simulink model "c09f12_01_avn"  (R2012b)
settings: Solver=ode45  StartTime=0.0  StopTime="(2^(7+2))  * (2^8)"  RelTol=1e-3
undefined symbols (not defined in the file): Down, pfb_coeff_gen_calc, Up, xlipgetpartsetting
libraries: xbsIndex_r4 x7041, casper_library_misc x193, xps_library x58, casper_library_delays x50, simulink x16, dspsigops x12, casper_library_flow_control x5, xbsReplacements_r4 x4, casper_library_ffts_twiddle x2, casper_library_multipliers x2, casper_library_reorder x1
(part 4 of 77)

== system c09f12_01_avn/decat0 ==
  In1 : Inport
  Reinterpret{1..4} (4 alike) : xbsIndex_r4/Reinterpret  force_arith_type=on  arith_type="Signed  (2's comp)"  force_bin_pt=on  bin_pt=0  block_type=reinterpret
      settings: infoedit="Changes signal type without altering the binary representation.   You can changed the signal between signed and unsigned, and relocate the binary point.<br><br>Hardware notes: In hardware this block costs nothing.<br><br>Example:  Suppose the input is 6 bits wide, signed, with 2 fractional bits, and the output is forced to unsigned with 0 fractional bits.  Then an input of -2.0 (1110.00 in binary 2's complement) becomes an output of 56 (111000 in binary)."  block_version=10.1.3
  Slice15 : xbsIndex_r4/Slice  nbits=8  boolean_output=off  mode=Lower Bit Location + Width  bit1=0  base1=MSB of Input  bit0=8  base0=LSB of Input  dbl_ovrd=off  block_type=slice
      settings: infoedit="Extracts a given range of bits from each input sample and presents it at the output.  The output type is ordinarily unsigned with binary point at zero, but can be Boolean when the slice is one bit wide.<P><P>Hardware notes: In hardware this block costs nothing."  block_version=10.1.3
  Slice16 : xbsIndex_r4/Slice  nbits=8  boolean_output=off  mode=Lower Bit Location + Width  bit1=0  base1=MSB of Input  bit0=16  base0=LSB of Input  dbl_ovrd=off  block_type=slice
      settings: infoedit="Extracts a given range of bits from each input sample and presents it at the output.  The output type is ordinarily unsigned with binary point at zero, but can be Boolean when the slice is one bit wide.<P><P>Hardware notes: In hardware this block costs nothing."  block_version=10.1.3
  Slice17 : xbsIndex_r4/Slice  nbits=8  boolean_output=off  mode=Lower Bit Location + Width  bit1=0  base1=MSB of Input  bit0=24  base0=LSB of Input  dbl_ovrd=off  block_type=slice
      settings: infoedit="Extracts a given range of bits from each input sample and presents it at the output.  The output type is ordinarily unsigned with binary point at zero, but can be Boolean when the slice is one bit wide.<P><P>Hardware notes: In hardware this block costs nothing."  block_version=10.1.3
  Slice9 : xbsIndex_r4/Slice  nbits=8  boolean_output=off  mode=Lower Bit Location + Width  bit1=0  base1=MSB of Input  bit0=0  base0=LSB of Input  dbl_ovrd=off  block_type=slice
      settings: infoedit="Extracts a given range of bits from each input sample and presents it at the output.  The output type is ordinarily unsigned with binary point at zero, but can be Boolean when the slice is one bit wide.<P><P>Hardware notes: In hardware this block costs nothing."  block_version=10.1.3
  Out1 : Outport
  Out2 : Outport  Port=2
  Out3 : Outport  Port=3
  Out4 : Outport  Port=4
  wires:
  Reinterpret4/1 -> Out4/1
  Reinterpret3/1 -> Out3/1
  Reinterpret1/1 -> Out2/1
  Reinterpret2/1 -> Out1/1
  Slice9/1 -> Reinterpret4/1
  Slice15/1 -> Reinterpret3/1
  Slice16/1 -> Reinterpret1/1
  Slice17/1 -> Reinterpret2/1
  In1/1 -> Slice15/1, Slice9/1, Slice16/1, Slice17/1

== system c09f12_01_avn/decat1 ==
  In1 : Inport
  Reinterpret{1..4} (4 alike) : xbsIndex_r4/Reinterpret  force_arith_type=on  arith_type="Signed  (2's comp)"  force_bin_pt=on  bin_pt=0  block_type=reinterpret
      settings: infoedit="Changes signal type without altering the binary representation.   You can changed the signal between signed and unsigned, and relocate the binary point.<br><br>Hardware notes: In hardware this block costs nothing.<br><br>Example:  Suppose the input is 6 bits wide, signed, with 2 fractional bits, and the output is forced to unsigned with 0 fractional bits.  Then an input of -2.0 (1110.00 in binary 2's complement) becomes an output of 56 (111000 in binary)."  block_version=10.1.3
  Slice15 : xbsIndex_r4/Slice  nbits=8  boolean_output=off  mode=Lower Bit Location + Width  bit1=0  base1=MSB of Input  bit0=8  base0=LSB of Input  dbl_ovrd=off  block_type=slice
      settings: infoedit="Extracts a given range of bits from each input sample and presents it at the output.  The output type is ordinarily unsigned with binary point at zero, but can be Boolean when the slice is one bit wide.<P><P>Hardware notes: In hardware this block costs nothing."  block_version=10.1.3
  Slice16 : xbsIndex_r4/Slice  nbits=8  boolean_output=off  mode=Lower Bit Location + Width  bit1=0  base1=MSB of Input  bit0=16  base0=LSB of Input  dbl_ovrd=off  block_type=slice
      settings: infoedit="Extracts a given range of bits from each input sample and presents it at the output.  The output type is ordinarily unsigned with binary point at zero, but can be Boolean when the slice is one bit wide.<P><P>Hardware notes: In hardware this block costs nothing."  block_version=10.1.3
  Slice17 : xbsIndex_r4/Slice  nbits=8  boolean_output=off  mode=Lower Bit Location + Width  bit1=0  base1=MSB of Input  bit0=24  base0=LSB of Input  dbl_ovrd=off  block_type=slice
      settings: infoedit="Extracts a given range of bits from each input sample and presents it at the output.  The output type is ordinarily unsigned with binary point at zero, but can be Boolean when the slice is one bit wide.<P><P>Hardware notes: In hardware this block costs nothing."  block_version=10.1.3
  Slice9 : xbsIndex_r4/Slice  nbits=8  boolean_output=off  mode=Lower Bit Location + Width  bit1=0  base1=MSB of Input  bit0=0  base0=LSB of Input  dbl_ovrd=off  block_type=slice
      settings: infoedit="Extracts a given range of bits from each input sample and presents it at the output.  The output type is ordinarily unsigned with binary point at zero, but can be Boolean when the slice is one bit wide.<P><P>Hardware notes: In hardware this block costs nothing."  block_version=10.1.3
  Out1 : Outport
  Out2 : Outport  Port=2
  Out3 : Outport  Port=3
  Out4 : Outport  Port=4
  wires:
  In1/1 -> Slice17/1, Slice16/1, Slice9/1, Slice15/1
  Slice17/1 -> Reinterpret2/1
  Slice16/1 -> Reinterpret1/1
  Slice15/1 -> Reinterpret3/1
  Slice9/1 -> Reinterpret4/1
  Reinterpret2/1 -> Out1/1
  Reinterpret1/1 -> Out2/1
  Reinterpret3/1 -> Out3/1
  Reinterpret4/1 -> Out4/1

== system c09f12_01_avn/delay_tr_status0 ==
  reg_out : Inport
  c09f12_01_avn_delay_tr_status0_user_data_in : xbsIndex_r4/Gateway Out  inherit_from_input=off  hdl_port=on  timing_constraint=None  locs_specified=off  LOCs={}  UseAsDAC=off  DACChannel='1'  block_type=gatewayout
  convert : xbsIndex_r4/Convert  gui_display_data_type=Fixed-point  arith_type=Unsigned  n_bits=32  bin_pt=0  float_type=Single  exp_bits=8  fraction_bits=24  quantization=Truncate  overflow=Wrap  en=off  latency=0  dbl_ovrd=off  pipeline=off  block_type=convert
  sim_reg_out : Outport
  wires:
  reg_out/1 -> convert/1
  convert/1 -> c09f12_01_avn_delay_tr_status0_user_data_in/1
  c09f12_01_avn_delay_tr_status0_user_data_in/1 -> sim_reg_out/1

== system c09f12_01_avn/delay_tr_status1 ==
  reg_out : Inport
  c09f12_01_avn_delay_tr_status1_user_data_in : xbsIndex_r4/Gateway Out  inherit_from_input=off  hdl_port=on  timing_constraint=None  locs_specified=off  LOCs={}  UseAsDAC=off  DACChannel='1'  block_type=gatewayout
  convert : xbsIndex_r4/Convert  gui_display_data_type=Fixed-point  arith_type=Unsigned  n_bits=32  bin_pt=0  float_type=Single  exp_bits=8  fraction_bits=24  quantization=Truncate  overflow=Wrap  en=off  latency=0  dbl_ovrd=off  pipeline=off  block_type=convert
  sim_reg_out : Outport
  wires:
  reg_out/1 -> convert/1
  convert/1 -> c09f12_01_avn_delay_tr_status1_user_data_in/1
  c09f12_01_avn_delay_tr_status1_user_data_in/1 -> sim_reg_out/1

== system c09f12_01_avn/edge_detect2 ==
  in : Inport
  Delay : xbsIndex_r4/Delay  rst=off  infoeditControl=Selection of Reset will increase slice count due to use of real FFs and instead of SRLs  en=off  latency=1  dbl_ovrd=off  reg_retiming=off  block_type=delay
      settings: xl_area=[0, 0, 0, 0, 0, 0, 0]
  Inverter : xbsIndex_r4/Inverter  en=off  latency=0  dbl_ovrd=off  block_type=inv
      settings: xl_area=[0, 0, 0, 0, 0, 0, 0]
  edge_op : xbsIndex_r4/Logical  logical_function=AND  inputs=2  en=off  latency=0  precision=Full  arith_type=Unsigned  n_bits=8  bin_pt=2  align_bp=on  dbl_ovrd=off  block_type=logical
      settings: xl_area=[0, 0, 0, 0, 0, 0, 0]
  out : Outport
  wires:
  Inverter/1 -> edge_op/1
  edge_op/1 -> out/1
  in/1 -> Inverter/1, Delay/1
  Delay/1 -> edge_op/2

== system c09f12_01_avn/eq0 ==
  addr : Inport
  data_in : Inport  Port=2
  we : Inport  Port=3
  c09f12_01_avn_eq0_addr : xbsIndex_r4/Gateway Out  inherit_from_input=off  hdl_port=on  timing_constraint=None  locs_specified=off  LOCs={'A5','B9','A9','C1','A3','G6','E9','A6','A7','A8','B8','B1','B3','D9','B5','B4','B6','C2'}  UseAsDAC=off  DACChannel='1'  block_type=gatewayout
      settings: infoedit="Gateway out block.  Converts Xilinx fixed point inputs into ouputs of type Simulink integer, double, or fixed point.<P><P>Hardware notes:  In hardware these blocks become top level output ports or are discarded, depending on how they are configured."  xl_area=[0, 0, 0, 0, 0, 0, 0]  sginterface={'Nallatech'=>{'xdspkit'=>{'non_memory_mapped_port'=>'uprev_Shared_BRAM_addr'}},'Xilinx'=>{'jtaghwcosim'=>{'non_memory_mapped_port'=>'uprev_Shared_BRAM_addr'},'xdspkit'=>{'non_memory_mapped_port'=>'uprev_Shared_BRAM_addr'}}}
  c09f12_01_avn_eq0_data_in : xbsIndex_r4/Gateway Out  inherit_from_input=off  hdl_port=on  timing_constraint=None  locs_specified=off  LOCs={'B21','B22','A22','B23','B19','C19','A20','A21','A23','B24','A24','A25','E18','D18','C18','B18'}  UseAsDAC=off  DACChannel='1'  block_type=gatewayout
      settings: infoedit="Gateway out block.  Converts Xilinx fixed point inputs into ouputs of type Simulink integer, double, or fixed point.<P><P>Hardware notes:  In hardware these blocks become top level output ports or are discarded, depending on how they are configured."  xl_area=[0, 0, 0, 0, 0, 0, 0]  sginterface={'Nallatech'=>{'xdspkit'=>{'non_memory_mapped_port'=>'uprev_Shared_BRAM_data_in'}},'Xilinx'=>{'jtaghwcosim'=>{'non_memory_mapped_port'=>'uprev_Shared_BRAM_data_in'},'xdspkit'=>{'non_memory_mapped_port'=>'uprev_Shared_BRAM_data_in'}}}
  c09f12_01_avn_eq0_data_out : xbsIndex_r4/Gateway In  gui_display_data_type=Fixed-point  arith_type=Unsigned  n_bits=data_width  bin_pt=data_bin_pt  preci_type=Single  exp_width=8  frac_width=24  quantization=Truncate  overflow=Wrap  period=sample_rate  dbl_ovrd=off  timing_constraint=None  locs_specified=off  LOCs={}  UseAsADC=off  ADCChannel='1'  inherit_from_input=off  hdl_port=on  block_type=gatewayin
      settings: infoedit="Gateway in block.  Converts inputs of type Simulink integer, double and fixed point to  Xilinx fixed point type.<br><br>Hardware notes:  In hardware these blocks become top level input ports."  xl_area=[0, 0, 0, 0, 0, 0, 0]
  c09f12_01_avn_eq0_we : xbsIndex_r4/Gateway Out  inherit_from_input=off  hdl_port=on  timing_constraint=None  locs_specified=off  LOCs={'A14'}  UseAsDAC=off  DACChannel='1'  block_type=gatewayout
      settings: infoedit="Gateway out block.  Converts Xilinx fixed point inputs into ouputs of type Simulink integer, double, or fixed point.<P><P>Hardware notes:  In hardware these blocks become top level output ports or are discarded, depending on how they are configured."  xl_area=[0, 0, 0, 0, 0, 0, 0]
  calc_add : Subsystem
  convert_addr : xbsIndex_r4/Convert  gui_display_data_type=Fixed-point  arith_type=Unsigned  n_bits=addr_width  bin_pt=0  float_type=Single  exp_bits=8  fraction_bits=24  quantization=Truncate  overflow=Wrap  en=off  latency=0  dbl_ovrd=off  pipeline=off  block_type=convert
      settings: xl_area=[0, 0, 0, 0, 0, 0, 0]
  convert_din : xbsIndex_r4/Convert  gui_display_data_type=Fixed-point  arith_type=Unsigned  n_bits=data_width  bin_pt=data_bin_pt  float_type=Single  exp_bits=8  fraction_bits=24  quantization=Truncate  overflow=Wrap  en=off  latency=0  dbl_ovrd=off  pipeline=off  block_type=convert
      settings: xl_area=[0, 0, 0, 0, 0, 0, 0]
  convert_din1 : xbsIndex_r4/Convert  gui_display_data_type=Fixed-point  arith_type=Unsigned  n_bits=data_width  bin_pt=data_bin_pt  float_type=Single  exp_bits=8  fraction_bits=24  quantization=Truncate  overflow=Wrap  en=off  latency=0  dbl_ovrd=off  pipeline=off  block_type=convert
      settings: xl_area=[0, 0, 0, 0, 0, 0, 0]
  convert_we : xbsIndex_r4/Convert  gui_display_data_type=Fixed-point  arith_type=Unsigned  n_bits=1  bin_pt=0  float_type=Single  exp_bits=8  fraction_bits=24  quantization=Truncate  overflow=Wrap  en=off  latency=0  dbl_ovrd=off  pipeline=off  block_type=convert
      settings: xl_area=[0, 0, 0, 0, 0, 0, 0]
  mem : Subsystem
  munge_in : Subsystem  AncestorBlock=casper_library_flow_control/munge  mask(munge){divisions=1, div_size=32, order=[0]}
      mask prompts: divisions "Number of divisions"; div_size "Division size (bits)"; order "Division packing order"
      mask help: Splits an input bus into the specified number of divisions and then recombines them in the order specified (most significant division = 0,least = number divisions-1)
      mask init:
      | munge_init(gcb, ...
      |     'divisions', divisions, ...
      |     'div_size', div_size, ...
      |     'order', order);
      settings: AttributesFormatString=|
      | [0]
      | 32 bits
  munge_out : Subsystem  AncestorBlock=casper_library_flow_control/munge  mask(munge){divisions=1, div_size=32, order=[0]}
      mask prompts: divisions "Number of divisions"; div_size "Division size (bits)"; order "Division packing order"
      mask help: Splits an input bus into the specified number of divisions and then recombines them in the order specified (most significant division = 0,least = number divisions-1)
      mask init:
      | munge_init(gcb, ...
      |     'divisions', divisions, ...
      |     'div_size', div_size, ...
      |     'order', order);
      settings: AttributesFormatString=|
      | [0]
      | 32 bits
  data_out : Outport
  wires:
  convert_din/1 -> munge_in/1(din)
  convert_din1/1 -> c09f12_01_avn_eq0_data_in/1
  convert_addr/1 -> c09f12_01_avn_eq0_addr/1
  calc_add/1(out) -> convert_addr/1
  munge_out/1(dout) -> data_out/1
  munge_in/1(dout) -> convert_din1/1
  c09f12_01_avn_eq0_we/1 -> mem/3(In3)
  c09f12_01_avn_eq0_data_in/1 -> mem/2(In2)
  c09f12_01_avn_eq0_addr/1 -> mem/1(In1)
  convert_we/1 -> c09f12_01_avn_eq0_we/1
  we/1 -> convert_we/1
  addr/1 -> calc_add/1(in)
  c09f12_01_avn_eq0_data_out/1 -> munge_out/1(din)
  data_in/1 -> convert_din/1
  mem/1(Out1) -> c09f12_01_avn_eq0_data_out/1

== system c09f12_01_avn/eq1 ==
  addr : Inport
  data_in : Inport  Port=2
  we : Inport  Port=3
  c09f12_01_avn_eq1_addr : xbsIndex_r4/Gateway Out  inherit_from_input=off  hdl_port=on  timing_constraint=None  locs_specified=off  LOCs={'A5','B9','A9','C1','A3','G6','E9','A6','A7','A8','B8','B1','B3','D9','B5','B4','B6','C2'}  UseAsDAC=off  DACChannel='1'  block_type=gatewayout
      settings: infoedit="Gateway out block.  Converts Xilinx fixed point inputs into ouputs of type Simulink integer, double, or fixed point.<P><P>Hardware notes:  In hardware these blocks become top level output ports or are discarded, depending on how they are configured."  xl_area=[0, 0, 0, 0, 0, 0, 0]  sginterface={'Nallatech'=>{'xdspkit'=>{'non_memory_mapped_port'=>'uprev_Shared_BRAM_addr'}},'Xilinx'=>{'jtaghwcosim'=>{'non_memory_mapped_port'=>'uprev_Shared_BRAM_addr'},'xdspkit'=>{'non_memory_mapped_port'=>'uprev_Shared_BRAM_addr'}}}
  c09f12_01_avn_eq1_data_in : xbsIndex_r4/Gateway Out  inherit_from_input=off  hdl_port=on  timing_constraint=None  locs_specified=off  LOCs={'B21','B22','A22','B23','B19','C19','A20','A21','A23','B24','A24','A25','E18','D18','C18','B18'}  UseAsDAC=off  DACChannel='1'  block_type=gatewayout
      settings: infoedit="Gateway out block.  Converts Xilinx fixed point inputs into ouputs of type Simulink integer, double, or fixed point.<P><P>Hardware notes:  In hardware these blocks become top level output ports or are discarded, depending on how they are configured."  xl_area=[0, 0, 0, 0, 0, 0, 0]  sginterface={'Nallatech'=>{'xdspkit'=>{'non_memory_mapped_port'=>'uprev_Shared_BRAM_data_in'}},'Xilinx'=>{'jtaghwcosim'=>{'non_memory_mapped_port'=>'uprev_Shared_BRAM_data_in'},'xdspkit'=>{'non_memory_mapped_port'=>'uprev_Shared_BRAM_data_in'}}}
  c09f12_01_avn_eq1_data_out : xbsIndex_r4/Gateway In  gui_display_data_type=Fixed-point  arith_type=Unsigned  n_bits=data_width  bin_pt=data_bin_pt  preci_type=Single  exp_width=8  frac_width=24  quantization=Truncate  overflow=Wrap  period=sample_rate  dbl_ovrd=off  timing_constraint=None  locs_specified=off  LOCs={}  UseAsADC=off  ADCChannel='1'  inherit_from_input=off  hdl_port=on  block_type=gatewayin
      settings: infoedit="Gateway in block.  Converts inputs of type Simulink integer, double and fixed point to  Xilinx fixed point type.<br><br>Hardware notes:  In hardware these blocks become top level input ports."  xl_area=[0, 0, 0, 0, 0, 0, 0]
  c09f12_01_avn_eq1_we : xbsIndex_r4/Gateway Out  inherit_from_input=off  hdl_port=on  timing_constraint=None  locs_specified=off  LOCs={'A14'}  UseAsDAC=off  DACChannel='1'  block_type=gatewayout
      settings: infoedit="Gateway out block.  Converts Xilinx fixed point inputs into ouputs of type Simulink integer, double, or fixed point.<P><P>Hardware notes:  In hardware these blocks become top level output ports or are discarded, depending on how they are configured."  xl_area=[0, 0, 0, 0, 0, 0, 0]
  calc_add : Subsystem
  convert_addr : xbsIndex_r4/Convert  gui_display_data_type=Fixed-point  arith_type=Unsigned  n_bits=addr_width  bin_pt=0  float_type=Single  exp_bits=8  fraction_bits=24  quantization=Truncate  overflow=Wrap  en=off  latency=0  dbl_ovrd=off  pipeline=off  block_type=convert
      settings: xl_area=[0, 0, 0, 0, 0, 0, 0]
  convert_din : xbsIndex_r4/Convert  gui_display_data_type=Fixed-point  arith_type=Unsigned  n_bits=data_width  bin_pt=data_bin_pt  float_type=Single  exp_bits=8  fraction_bits=24  quantization=Truncate  overflow=Wrap  en=off  latency=0  dbl_ovrd=off  pipeline=off  block_type=convert
      settings: xl_area=[0, 0, 0, 0, 0, 0, 0]
  convert_din1 : xbsIndex_r4/Convert  gui_display_data_type=Fixed-point  arith_type=Unsigned  n_bits=data_width  bin_pt=data_bin_pt  float_type=Single  exp_bits=8  fraction_bits=24  quantization=Truncate  overflow=Wrap  en=off  latency=0  dbl_ovrd=off  pipeline=off  block_type=convert
      settings: xl_area=[0, 0, 0, 0, 0, 0, 0]
  convert_we : xbsIndex_r4/Convert  gui_display_data_type=Fixed-point  arith_type=Unsigned  n_bits=1  bin_pt=0  float_type=Single  exp_bits=8  fraction_bits=24  quantization=Truncate  overflow=Wrap  en=off  latency=0  dbl_ovrd=off  pipeline=off  block_type=convert
      settings: xl_area=[0, 0, 0, 0, 0, 0, 0]
  mem : Subsystem
  munge_in : Subsystem  AncestorBlock=casper_library_flow_control/munge  mask(munge){divisions=1, div_size=32, order=[0]}
      mask prompts: divisions "Number of divisions"; div_size "Division size (bits)"; order "Division packing order"
      mask help: Splits an input bus into the specified number of divisions and then recombines them in the order specified (most significant division = 0,least = number divisions-1)
      mask init:
      | munge_init(gcb, ...
      |     'divisions', divisions, ...
      |     'div_size', div_size, ...
      |     'order', order);
      settings: AttributesFormatString=|
      | [0]
      | 32 bits
  munge_out : Subsystem  AncestorBlock=casper_library_flow_control/munge  mask(munge){divisions=1, div_size=32, order=[0]}
      mask prompts: divisions "Number of divisions"; div_size "Division size (bits)"; order "Division packing order"
      mask help: Splits an input bus into the specified number of divisions and then recombines them in the order specified (most significant division = 0,least = number divisions-1)
      mask init:
      | munge_init(gcb, ...
      |     'divisions', divisions, ...
      |     'div_size', div_size, ...
      |     'order', order);
      settings: AttributesFormatString=|
      | [0]
      | 32 bits
  data_out : Outport
  wires:
  convert_din/1 -> munge_in/1(din)
  convert_din1/1 -> c09f12_01_avn_eq1_data_in/1
  convert_addr/1 -> c09f12_01_avn_eq1_addr/1
  calc_add/1(out) -> convert_addr/1
  munge_out/1(dout) -> data_out/1
  munge_in/1(dout) -> convert_din1/1
  c09f12_01_avn_eq1_we/1 -> mem/3(In3)
  c09f12_01_avn_eq1_data_in/1 -> mem/2(In2)
  c09f12_01_avn_eq1_addr/1 -> mem/1(In1)
  convert_we/1 -> c09f12_01_avn_eq1_we/1
  we/1 -> convert_we/1
  addr/1 -> calc_add/1(in)
  c09f12_01_avn_eq1_data_out/1 -> munge_out/1(din)
  data_in/1 -> convert_din/1
  mem/1(Out1) -> c09f12_01_avn_eq1_data_out/1

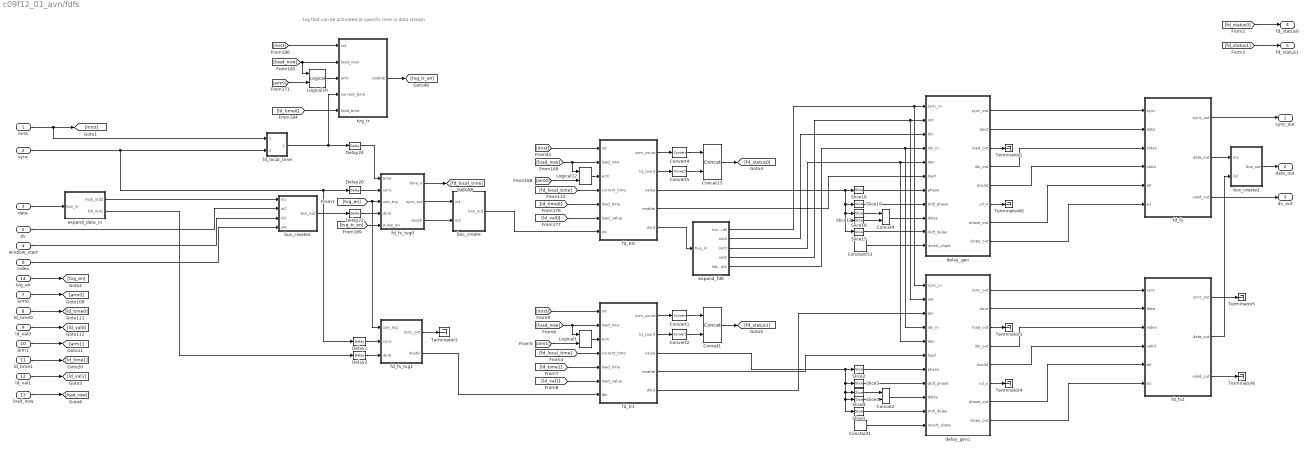
== system c09f12_01_avn/fdfs ==
  note: tvg that can be activated at
      | specific time in data stream
  mrst : Inport
  sync : Inport  Port=2
  data : Inport  Port=3
  window_start : Inport  Port=4
  dv : Inport  Port=5
  index : Inport  Port=6
  arm0 : Inport  Port=7
  ld_time0 : Inport  Port=8
  ld_val0 : Inport  Port=9
  arm1 : Inport  Port=10
  ld_time1 : Inport  Port=11
  ld_val1 : Inport  Port=12
  load_now : Inport  Port=13
  tvg_en : Inport  Port=14
  Concat{1..2,4,13} (4 alike) : xbsIndex_r4/Concat  num_inputs=2  dbl_ovrd=off  block_type=concat
      Concat1 settings: block_version=10.1.3
      Concat13 settings: block_version=10.1.3
  Constant1 : xbsIndex_r4/Constant  const=0  gui_display_data_type=Fixed-point  arith_type=Boolean  n_bits=1  bin_pt=0  preci_type=Single  exp_width=8  frac_width=24  explicit_period=off  period=1  equ=P=C  opselect=C  inp2=PCIN>>17  opr=+  inp1=P  carry=CIN  dbl_ovrd=off  block_type=constant
      settings: block_version=11.4
  Constant53 : xbsIndex_r4/Constant  const=0  gui_display_data_type=Fixed-point  arith_type=Boolean  n_bits=1  bin_pt=0  preci_type=Single  exp_width=8  frac_width=24  explicit_period=off  period=1  equ=P=C  opselect=C  inp2=PCIN>>17  opr=+  inp1=P  carry=CIN  dbl_ovrd=off  block_type=constant
      settings: block_version=11.4
  Convert{1..2,4..5} (4 alike) : xbsIndex_r4/Convert  gui_display_data_type=Fixed-point  arith_type=Unsigned  n_bits=16  bin_pt=0  float_type=Single  exp_bits=8  fraction_bits=24  quantization=Truncate  overflow=Wrap  en=off  latency=0  dbl_ovrd=off  pipeline=on  block_type=convert
      settings: block_version=11.4
  Delay{1..2,20,22,24} (5 alike) : xbsIndex_r4/Delay  rst=off  infoeditControl=Selection of Reset will increase slice count due to use of real FFs and instead of SRLs  en=off  latency=4  dbl_ovrd=off  reg_retiming=off  block_type=delay
      settings: block_version=11.4
  Logical1 : xbsIndex_r4/Logical  logical_function=OR  inputs=2  en=off  latency=0  precision=Full  arith_type=Unsigned  n_bits=16  bin_pt=0  align_bp=on  dbl_ovrd=off  block_type=logical
      settings: block_version=11.4
  Logical12 : xbsIndex_r4/Logical  logical_function=OR  inputs=2  en=off  latency=0  precision=Full  arith_type=Unsigned  n_bits=16  bin_pt=0  align_bp=on  dbl_ovrd=off  block_type=logical
      settings: block_version=11.4
  Logical20 : xbsIndex_r4/Logical  logical_function=OR  inputs=2  en=off  latency=0  precision=Full  arith_type=Unsigned  n_bits=16  bin_pt=0  align_bp=on  dbl_ovrd=off  block_type=logical
      settings: block_version=11.4
  Slice1 : xbsIndex_r4/Slice  nbits=16  boolean_output=off  mode=Lower Bit Location + Width  bit1=0  base1=MSB of Input  bit0=0*16  base0=LSB of Input  dbl_ovrd=off  block_type=slice
      settings: block_version=10.1.3
  Slice15 : xbsIndex_r4/Slice  nbits=16  boolean_output=off  mode=Lower Bit Location + Width  bit1=0  base1=MSB of Input  bit0=0*16  base0=LSB of Input  dbl_ovrd=off  block_type=slice
      settings: block_version=10.1.3
  Slice16 : xbsIndex_r4/Slice  nbits=16  boolean_output=off  mode=Lower Bit Location + Width  bit1=0  base1=MSB of Input  bit0=16*3+15  base0=LSB of Input  dbl_ovrd=off  block_type=slice
      settings: block_version=10.1.3
  Slice17 : xbsIndex_r4/Slice  nbits=16  boolean_output=off  mode=Lower Bit Location + Width  bit1=0  base1=MSB of Input  bit0=16*1  base0=LSB of Input  dbl_ovrd=off  block_type=slice
      settings: block_version=10.1.3
  Slice18 : xbsIndex_r4/Slice  nbits=15  boolean_output=off  mode=Lower Bit Location + Width  bit1=0  base1=MSB of Input  bit0=16*2  base0=LSB of Input  dbl_ovrd=off  block_type=slice
      settings: block_version=10.1.3
  Slice19 : xbsIndex_r4/Slice  nbits=16  boolean_output=off  mode=Lower Bit Location + Width  bit1=0  base1=MSB of Input  bit0=16*2+15  base0=LSB of Input  dbl_ovrd=off  block_type=slice
      settings: block_version=10.1.3
  Slice2 : xbsIndex_r4/Slice  nbits=16  boolean_output=off  mode=Lower Bit Location + Width  bit1=0  base1=MSB of Input  bit0=16*3+15  base0=LSB of Input  dbl_ovrd=off  block_type=slice
      settings: block_version=10.1.3
  Slice3 : xbsIndex_r4/Slice  nbits=16  boolean_output=off  mode=Lower Bit Location + Width  bit1=0  base1=MSB of Input  bit0=16*1  base0=LSB of Input  dbl_ovrd=off  block_type=slice
      settings: block_version=10.1.3
  Slice4 : xbsIndex_r4/Slice  nbits=15  boolean_output=off  mode=Lower Bit Location + Width  bit1=0  base1=MSB of Input  bit0=16*2  base0=LSB of Input  dbl_ovrd=off  block_type=slice
      settings: block_version=10.1.3
  Slice5 : xbsIndex_r4/Slice  nbits=16  boolean_output=off  mode=Lower Bit Location + Width  bit1=0  base1=MSB of Input  bit0=16*2+15  base0=LSB of Input  dbl_ovrd=off  block_type=slice
      settings: block_version=10.1.3
  Terminator{1..6,60} (7 alike) : Terminator
  bus_create : Subsystem  AncestorBlock=casper_library_flow_control/bus_create  mask(bus_create){inputNum=2}
      mask prompts: inputNum "Number of inputs:"
      mask init:
      | bus_create_init(gcb,...
      |     'inputNum', inputNum);
  bus_create1 : Subsystem  AncestorBlock=casper_library_flow_control/bus_create  mask(bus_create){inputNum=2}
      mask prompts: inputNum "Number of inputs:"
      mask init:
      | bus_create_init(gcb,...
      |     'inputNum', inputNum);
  bus_create2 : Subsystem  AncestorBlock=casper_library_flow_control/bus_create  mask(bus_create){inputNum=4}
      mask prompts: inputNum "Number of inputs:"
      mask init:
      | bus_create_init(gcb,...
      |     'inputNum', inputNum);
  delay_gen : Subsystem  mask{fft_len=coarse_fft_bits - 1 + fine_fft_bits, phase_bits=16, max_fringe_rate=23, min_fringe_rate=38, delay_bits=16+15, delay_bin_pt=16, max_delay_rate=23, min_delay_rate=38, add_latency=1, lookup_bits=11, cd_bits=13, data_bits=data_bits * 2}
      mask prompts: fft_len "FFT size (2^?)"; phase_bits "Input phase resolution (2*pi/2^? radians)"; max_fringe_rate "Max fringe update rate (1/2^? radians/sample)"; min_fringe_rate "Min (non-zero) fringe rate (1/2^? radians/sample)"; delay_bits "Input delay resolution (bits)"; delay_bin_pt "Input delay binary point"; max_delay_rate "Max delay update rate (1/2^? samples/sample)"; min_delay_rate "Min (non-zero) delay update rate (1/2^? samples/sample)"; add_latency "Add latency"; lookup_bits "DDS lookup table resolution (2*pi/2^?)"; cd_bits "Coarse delay range (2^? bits)"; data_bits "Data width"
  delay_gen1 : Subsystem  mask{fft_len=coarse_fft_bits - 1 + fine_fft_bits, phase_bits=16, max_fringe_rate=23, min_fringe_rate=38, delay_bits=16+15, delay_bin_pt=16, max_delay_rate=23, min_delay_rate=38, add_latency=1, lookup_bits=11, cd_bits=13, data_bits=data_bits * 2}
      mask prompts: fft_len "FFT size (2^?)"; phase_bits "Input phase resolution (2*pi/2^? radians)"; max_fringe_rate "Max fringe update rate (1/2^? radians/sample)"; min_fringe_rate "Min (non-zero) fringe rate (1/2^? radians/sample)"; delay_bits "Input delay resolution (bits)"; delay_bin_pt "Input delay binary point"; max_delay_rate "Max delay update rate (1/2^? samples/sample)"; min_delay_rate "Min (non-zero) delay update rate (1/2^? samples/sample)"; add_latency "Add latency"; lookup_bits "DDS lookup table resolution (2*pi/2^?)"; cd_bits "Coarse delay range (2^? bits)"; data_bits "Data width"
  expand_data_in : Subsystem  AncestorBlock=casper_library_flow_control/bus_expand  mask(bus_expand){mode=divisions of equal size, outputNum=2, outputWidth=data_bits*2, outputBinaryPt=0, outputArithmeticType=0, show_format=on, outputToWorkspace=off, variablePrefix=out, outputToModelAsWell=on}
      mask prompts: outputNum "Number of outputs:"; outputWidth "Output width:"; outputBinaryPt "Output binary point position:"; outputArithmeticType "Output arithmetic type: (Unsigned=0, Signed=1, Boolean=2)"; show_format "Print format string?"; outputToWorkspace "Output to workspace?"; variablePrefix "Variable name prefix:"; outputToModelAsWell "Output to model as well?"
      mask help:
      | Expands a 'bus' made using a bus_create or Xilinx
      | concat block.
      | The input will be divided into the specified number
      | of outputs with the specified arithmetic types.
      | Divisions are made from most significant bit.
      mask init: same as c09f12_01_avn/bus_expand6
      settings: AttributesFormatString=2 outputs: uf62.0,uf62.0,
      mask TypeOptions mode: divisions of equal size | divisions of arbitrary size
      mask Callback mode: bus_expand_callback();
      mask Callback outputWidth: bus_expand_callback();
      mask Callback outputToWorkspace: bus_expand_callback();
  expand_fd0 : Subsystem  AncestorBlock=casper_library_flow_control/bus_expand  mask(bus_expand){mode=divisions of arbitrary size, outputNum=5, outputWidth=getfield( getfield( get_param( gcb,'UserData' ), 'parameters'),'outputWidth'), outputBinaryPt=getfield( getfield( get_param( gcb,'UserData' ), 'parameters'),'outputBinaryPt'), outputArithmeticType=getfield( getfield( get_param( gcb,'UserData' ), 'parameters'),'outputArithmeticType'), show_format=on, outputToWorkspace=off, variablePrefix=out, outputToModelAsWell=on}
      mask prompts: outputNum "Number of outputs:"; outputWidth "Output width:"; outputBinaryPt "Output binary point position:"; outputArithmeticType "Output arithmetic type: (Unsigned=0, Signed=1, Boolean=2)"; show_format "Print format string?"; outputToWorkspace "Output to workspace?"; variablePrefix "Variable name prefix:"; outputToModelAsWell "Output to model as well?"
      mask help:
      | Expands a 'bus' made using a bus_create or Xilinx
      | concat block.
      | The input will be divided into the specified number
      | of outputs with the specified arithmetic types.
      | Divisions are made from most significant bit.
      mask init: same as c09f12_01_avn/bus_expand6
      settings: AttributesFormatString=5 outputs: b,uf62.0,b,b,uf20.0,
      mask TypeOptions mode: divisions of equal size | divisions of arbitrary size
      mask Callback mode: bus_expand_callback();
      mask Callback outputWidth: bus_expand_callback();
      mask Callback outputToWorkspace: bus_expand_callback();
  fd_fs : Subsystem  mask{lookup_bit_width=10, data_bit_width=data_bits, data_bp=data_bp, fft_len=coarse_fft_bits - 1 + fine_fft_bits, mix_bits=18, bram_latency=3, mult_latency=3, add_latency=2, conv_latency=2}
      mask prompts: lookup_bit_width "Phase resolution (2pi/2^?)"; data_bit_width "Data bit width"; data_bp "Data binary pt:"; fft_len "FFT length 2^?"; mix_bits "Mixing product bit width"; bram_latency "BRAM latency"; mult_latency "Mult latency"; add_latency "Adder latency"; conv_latency "Convert latency"
      mask init:
      | set_param([gcb,'/sincos0'], ...
      |     'bit_width', 'mix_bits', ...
      |     'bram_latency', 'bram_latency', ...
      |     'depth_bits', 'lookup_bit_width');
  fd_fs1 : Subsystem  mask{lookup_bit_width=10, data_bit_width=data_bits, data_bp=data_bp, fft_len=coarse_fft_bits - 1 + fine_fft_bits, mix_bits=18, bram_latency=3, mult_latency=3, add_latency=2, conv_latency=2}
      mask prompts: lookup_bit_width "Phase resolution (2pi/2^?)"; data_bit_width "Data bit width"; data_bp "Data binary pt:"; fft_len "FFT length 2^?"; mix_bits "Mixing product bit width"; bram_latency "BRAM latency"; mult_latency "Mult latency"; add_latency "Adder latency"; conv_latency "Convert latency"
      mask init:
      | set_param([gcb,'/sincos0'], ...
      |     'bit_width', 'mix_bits', ...
      |     'bram_latency', 'bram_latency', ...
      |     'depth_bits', 'lookup_bit_width');
  fd_fs_tvg0 : Subsystem  mask{bit_width=data_bits, bin_pt=data_bp, constant=1/16}
      mask prompts: bit_width "bit width"; bin_pt "binary point"
  fd_fs_tvg1 : Subsystem  mask{bit_width=data_bits, bin_pt=data_bp, val=1/16}
      mask prompts: bit_width "bit width"; bin_pt "binary point"; val "constant"
  fd_local_time : Subsystem
  fd_tr0 : Subsystem  mask{cnt_bits=8, time_bits=48}
      mask prompts: cnt_bits "Bits in status counters"; time_bits "No LSBs in time to compare"
  fd_tr1 : Subsystem  mask{cnt_bits=8, time_bits=48}
      mask prompts: cnt_bits "Bits in status counters"; time_bits "No LSBs in time to compare"
  tvg_tr : Subsystem  mask{cnt_bits=8, time_bits=48}
      mask prompts: cnt_bits "Bits in status counters"; time_bits "No LSBs in time to compare"
  sync_out : Outport
  data_out : Outport  Port=2
  dv_out : Outport  Port=3
  fd_status0 : Outport  Port=4
  fd_status1 : Outport  Port=5
  wires:
  data/1 -> expand_data_in/1(bus_in)
  fd_local_time/1(time) -> Delay24/1, tvg_tr/4(current_time)
  [mrst] -> fd_tr0/1(rst)
  Logical12/1 -> fd_tr0/3(arm)
  [fd_local_time] -> fd_tr0/4(current_time)
  [arm0] -> Logical12/2
  [load_now] -> Logical12/1, fd_tr0/2(load_now)
  fd_tr0/1(arm_count) -> Convert4/1
  fd_tr0/2(ld_count) -> Convert5/1
  [ld_time0] -> fd_tr0/5(load_time)
  [ld_val0] -> fd_tr0/6(load_value)
  fd_tr0/5(dout) -> expand_fd0/1(bus_in)
  fd_fs_tvg0/3(dout0) -> bus_create/2(in2)
  fd_fs_tvg0/2(sync_out) -> bus_create/1(in1)
  fd_fs_tvg0/1(time_o) -> [fd_local_time]
  [mrst] -> tvg_tr/1(rst)
  Logical20/1 -> tvg_tr/3(arm)
  [arm0] -> Logical20/2
  [load_now] -> tvg_tr/2(load_now), Logical20/1
  [ld_time0] -> tvg_tr/5(load_time)
  tvg_tr/1(enable) -> [tvg_tr_en]
  Delay20/1 -> fd_fs_tvg0/2(sync)
  Delay22/1 -> fd_fs_tvg0/4(din0)
  Delay24/1 -> fd_fs_tvg0/1(time)
  [tvg_tr_en] -> fd_fs_tvg0/5(pulse_en)
  Convert4/1 -> Concat13/1
  Concat13/1 -> [fd_status0]
  Convert5/1 -> Concat13/2
  sync/1 -> fd_local_time/2(sync), Delay20/1, Delay1/1
  Delay2/1 -> fd_fs_tvg1/3(din0)
  mrst/1 -> fd_local_time/1(reset), [mrst]
  Delay1/1 -> fd_fs_tvg1/2(sync)
  tvg_en/1 -> [tvg_en]
  [tvg_en] -> fd_fs_tvg0/3(use_tvg), fd_fs_tvg1/1(use_tvg)
  expand_data_in/1(msb_out2) -> bus_create2/1(in1)
  expand_data_in/2(lsb_out1) -> Delay2/1
  bus_create2/1(bus_out) -> Delay22/1
  fd_fs_tvg1/1(sync_out) -> Terminator2/1
  bus_create/1(bus_out) -> fd_tr0/7(din)
  arm0/1 -> [arm0]
  ld_time0/1 -> [ld_time0]
  ld_val0/1 -> [ld_val0]
  arm1/1 -> [arm1]
  ld_time1/1 -> [ld_time1]
  ld_val1/1 -> [ld_val1]
  dv/1 -> bus_create2/2(in2)
  window_start/1 -> bus_create2/3(in3)
  index/1 -> bus_create2/4(in4)
  [fd_status0] -> fd_status0/1
  [fd_status1] -> fd_status1/1
  [mrst] -> fd_tr1/1(rst)
  Logical1/1 -> fd_tr1/3(arm)
  [fd_local_time] -> fd_tr1/4(current_time)
  [arm1] -> Logical1/2
  [load_now] -> fd_tr1/2(load_now), Logical1/1
  fd_tr1/1(arm_count) -> Convert1/1
  fd_tr1/2(ld_count) -> Convert2/1
  [ld_time1] -> fd_tr1/5(load_time)
  [ld_val1] -> fd_tr1/6(load_value)
  Convert1/1 -> Concat1/1
  Concat1/1 -> [fd_status1]
  Convert2/1 -> Concat1/2
  fd_fs_tvg1/2(dout0) -> fd_tr1/7(din)
  Concat4/1 -> delay_gen/9(delay)
  Constant53/1 -> delay_gen/11(invert_slope)
  delay_gen/1(sync_out) -> fd_fs/1(sync)
  delay_gen/2(dout) -> fd_fs/2(data)
  delay_gen/3(load_out) -> Terminator1/1
  delay_gen/6(cd_o) -> Terminator60/1
  delay_gen/4(idx_out) -> fd_fs/3(index)
  delay_gen/5(dvalid) -> fd_fs/4(valid)
  delay_gen/7(phase_out) -> fd_fs/5(a0)
  delay_gen/8(slope_out) -> fd_fs/6(a1)
  fd_tr0/3(value) -> Slice16/1, Slice19/1, Slice18/1, Slice15/1, Slice17/1
  Slice16/1 -> delay_gen/7(phase)
  Slice19/1 -> delay_gen/8(d/dt_phase)
  Slice18/1 -> Concat4/1
  Slice17/1 -> Concat4/2
  Slice15/1 -> delay_gen/10(d/dt_delay)
  fd_fs/1(sync_out) -> sync_out/1
  fd_fs/3(valid_out) -> dv_out/1
  expand_fd0/1(msb_out5) -> delay_gen/1(sync_in), delay_gen1/1(sync_in)
  expand_fd0/2(out4) -> delay_gen/3(din)
  expand_fd0/3(out3) -> delay_gen/5(den), delay_gen1/5(den)
  expand_fd0/4(out2) -> delay_gen/2(init), delay_gen1/2(init)
  expand_fd0/5(lsb_out1) -> delay_gen/4(idx_in), delay_gen1/4(idx_in)
  fd_tr0/4(enable) -> delay_gen/6(load)
  Concat2/1 -> delay_gen1/9(delay)
  Constant1/1 -> delay_gen1/11(invert_slope)
  delay_gen1/1(sync_out) -> fd_fs1/1(sync)
  delay_gen1/2(dout) -> fd_fs1/2(data)
  delay_gen1/3(load_out) -> Terminator3/1
  delay_gen1/6(cd_o) -> Terminator4/1
  delay_gen1/4(idx_out) -> fd_fs1/3(index)
  delay_gen1/5(dvalid) -> fd_fs1/4(valid)
  delay_gen1/7(phase_out) -> fd_fs1/5(a0)
  delay_gen1/8(slope_out) -> fd_fs1/6(a1)
  Slice2/1 -> delay_gen1/7(phase)
  Slice5/1 -> delay_gen1/8(d/dt_phase)
  Slice4/1 -> Concat2/1
  Slice3/1 -> Concat2/2
  Slice1/1 -> delay_gen1/10(d/dt_delay)
  fd_tr1/3(value) -> Slice2/1, Slice5/1, Slice4/1, Slice1/1, Slice3/1
  fd_tr1/5(dout) -> delay_gen1/3(din)
  fd_tr1/4(enable) -> delay_gen1/6(load)
  fd_fs/2(data_out) -> bus_create1/1(in1)
  bus_create1/1(bus_out) -> data_out/1
  fd_fs1/2(data_out) -> bus_create1/2(in2)
  fd_fs1/1(sync_out) -> Terminator5/1
  fd_fs1/3(valid_out) -> Terminator6/1
  load_now/1 -> [load_now]

== system c09f12_01_avn/fine ==
  note: Output has one extra delay.
  sync : Inport
  data : Inport  Port=2
  coarse_chan_sel : Inport  Port=3
  fine_fft_shift : Inport  Port=4
  tvg_en : Inport  Port=5
  mrst : Inport  Port=6
  Concat2 : xbsIndex_r4/Concat  num_inputs=2  dbl_ovrd=off  block_type=concat
  Convert1 : xbsIndex_r4/Convert  gui_display_data_type=Fixed-point  arith_type=Unsigned  n_bits=64  bin_pt=0  float_type=Single  exp_bits=8  fraction_bits=24  quantization=Truncate  overflow=Wrap  en=off  latency=0  dbl_ovrd=off  pipeline=off  block_type=convert
      settings: block_version=11.4
  Convert2 : xbsIndex_r4/Convert  gui_display_data_type=Fixed-point  arith_type=Unsigned  n_bits=64  bin_pt=0  float_type=Single  exp_bits=8  fraction_bits=24  quantization=Truncate  overflow=Wrap  en=off  latency=0  dbl_ovrd=off  pipeline=off  block_type=convert
      settings: block_version=11.4
  Convert6 : xbsIndex_r4/Convert  gui_display_data_type=Fixed-point  arith_type=Unsigned  n_bits=128  bin_pt=0  float_type=Single  exp_bits=8  fraction_bits=24  quantization=Truncate  overflow=Wrap  en=off  latency=0  dbl_ovrd=off  pipeline=off  block_type=convert
      settings: block_version=11.4
  Delay1 : xbsIndex_r4/Delay  rst=off  infoeditControl=Selection of Reset will increase slice count due to use of real FFs and instead of SRLs  en=off  latency=2  dbl_ovrd=off  reg_retiming=on  block_type=delay
      settings: block_version=11.4
  Delay2 : xbsIndex_r4/Delay  rst=off  infoeditControl=Selection of Reset will increase slice count due to use of real FFs and instead of SRLs  en=off  latency=1  dbl_ovrd=off  reg_retiming=on  block_type=delay
      settings: block_version=11.4
  Delay4 : xbsIndex_r4/Delay  rst=off  infoeditControl=Selection of Reset will increase slice count due to use of real FFs and instead of SRLs  en=off  latency=2  dbl_ovrd=off  reg_retiming=on  block_type=delay
      settings: block_version=11.4
  Delay5 : xbsIndex_r4/Delay  rst=off  infoeditControl=Selection of Reset will increase slice count due to use of real FFs and instead of SRLs  en=off  latency=2  dbl_ovrd=off  reg_retiming=on  block_type=delay
      settings: block_version=11.4
  Delay6 : xbsIndex_r4/Delay  rst=off  infoeditControl=Selection of Reset will increase slice count due to use of real FFs and instead of SRLs  en=off  latency=1  dbl_ovrd=off  reg_retiming=on  block_type=delay
      settings: block_version=11.4
  Mux4 : xbsIndex_r4/Mux  inputs=2  en=off  latency=1  precision=Full  arith_type=Unsigned  n_bits=16  bin_pt=14  quantization=Truncate  overflow=Wrap  dbl_ovrd=off  block_type=mux
      settings: block_version=11.4
  buffer : Subsystem  mask{coarse_fft_bits=coarse_chan_bits, par_in=parallel_coarse_streams, fine_fft_bits=fine_fft_bits, bitwidth=36}
      mask prompts: coarse_fft_bits "Coarse FFT points (2^?):"; par_in "Parallel streams (2^?):"; fine_fft_bits "Fine FFT bits (2^?):"; bitwidth "Complex word bitwidth:"
  bus_create : casper_library_flow_control/bus_create  inputNum=2
  bus_create1 : Subsystem  AncestorBlock=casper_library_flow_control/bus_create  mask(bus_create){inputNum=3}
      mask prompts: inputNum "Number of inputs:"
      mask init:
      | bus_create_init(gcb,...
      |     'inputNum', inputNum);
  bus_create2 : Subsystem  AncestorBlock=casper_library_flow_control/bus_create  mask(bus_create){inputNum=3}
      mask prompts: inputNum "Number of inputs:"
      mask init:
      | bus_create_init(gcb,...
      |     'inputNum', inputNum);
  bus_create3 : Subsystem  AncestorBlock=casper_library_flow_control/bus_create  mask(bus_create){inputNum=3}
      mask prompts: inputNum "Number of inputs:"
      mask init:
      | bus_create_init(gcb,...
      |     'inputNum', inputNum);
  bus_expand1 : Subsystem  AncestorBlock=casper_library_flow_control/bus_expand  mask(bus_expand){mode=divisions of equal size, outputNum=2, outputWidth=36, outputBinaryPt=0, outputArithmeticType=0, show_format=on, outputToWorkspace=off, variablePrefix=out, outputToModelAsWell=on}
      mask prompts: outputNum "Number of outputs:"; outputWidth "Output width:"; outputBinaryPt "Output binary point position:"; outputArithmeticType "Output arithmetic type: (Unsigned=0, Signed=1, Boolean=2)"; show_format "Print format string?"; outputToWorkspace "Output to workspace?"; variablePrefix "Variable name prefix:"; outputToModelAsWell "Output to model as well?"
      mask help:
      | Expands a 'bus' made using a bus_create or Xilinx
      | concat block.
      | The input will be divided into the specified number
      | of outputs with the specified arithmetic types.
      | Divisions are made from most significant bit.
      mask init: same as c09f12_01_avn/bus_expand6
      settings: AttributesFormatString=2 outputs: uf36.0,uf36.0,
      mask TypeOptions mode: divisions of equal size | divisions of arbitrary size
      mask Callback mode: bus_expand_callback();
      mask Callback outputWidth: bus_expand_callback();
      mask Callback outputToWorkspace: bus_expand_callback();
  indexgen : Subsystem  mask{c_bits=coarse_chan_bits, f_bits=fine_fft_bits}
      mask prompts: c_bits "Coarse chans (2^?):"; f_bits "Fine chans (2^?):"
  pfb_fir_async1 : Subsystem  AncestorBlock=casper_library_pfbs/pfb_fir_async  mask(pfb_fir_async){pfb_bits=12, total_taps=2, window_type=hamming, simul_bits=1, make_biplex=off, data_in_bits=8, data_out_bits=18, coeff_bits=8, coeffs_in_distmem=off, add_latency=2, mult_latency=3, bram_latency=3, fan_latency=1, quantization=Truncate, fwidth=1, mult_spec=2, coeffs_share=off, async=on, debug_mode=off}
      mask prompts: pfb_bits "Size of PFB: (2^? pnts)"; total_taps "Total Number of Taps:"; window_type "Windowing Function:"; simul_bits "Number of Simultaneous Inputs: (2^?)"; make_biplex "Make Biplex?"; data_in_bits "Input Bitwidth:"; data_out_bits "Output Bitwidth:"; coeff_bits "Coefficient Bitwidth:"; coeffs_in_distmem "Use distributed memory for coeffs"; add_latency "Add Latency"; mult_latency "Mult Latency"; bram_latency "BRAM Latency"; fan_latency "Fanout latency"; quantization "Quantization Behavior"; fwidth "Bin Width Scaling (normal=1)"; mult_spec "Multiplier specification (0=core, 1=embedded, 2=behavioural) (left=1st tap, or just one value)"; coeffs_share "Share coefficients between polarisations (use less BRAM)?"; async "Make asynchronous"; debug_mode "Debug mode - coeffs are a [1:pfb_size*taps] ramp."
      mask init:
      | pfb_fir_async_init(gcb, ...
      |     'pfb_bits', pfb_bits, ...
      |     'total_taps', total_taps, ...
      |     'window_type', window_type, ...
      |     'simul_bits', simul_bits, ...
      |     'make_biplex', make_biplex, ...
      |     'data_in_bits', data_in_bits, ...
      |     'data_out_bits', data_out_bits, ...
      |     'coeff_bits', coeff_bits, ...
      |     'coeffs_in_distmem', coeffs_in_distmem, ...
      |     'add_latency', add_latency, ...
      |     'mult_latency', mult_latency, ...
      |     'bram_latency', bram_latency, ...
      |     'fan_latency', fan_latency, ...
      |     'quantization', quantization, ...
      |     'fwidth', fwidth, ...
      |     'mult_spec', mult_spec, ...
      |     'coeffs_share', coeffs_share, ...
      |     'async', async, ...
      |     'debug_mode', debug_mode);
      settings: AttributesFormatString=|
      | taps=2, add_latency=2
      | max scale 0.500
      mask Help: eval('xlWeb(''http://casper.berkeley.edu/wiki/Pfb_fir'')')
      mask TypeOptions window_type: bartlett | barthannwin | blackman | blackmanharris | bohamwin | chebwin | flattopwin | gausswin | hamming | hann | kaiser | nuttallwin | parzenwin | rectwin | tukeywin | triang | userwindow
      mask TypeOptions quantization: Truncate | Round  (unbiased: +/- Inf) | Round  (unbiased: Even Values)
  xilinx_ffts : Subsystem  mask{coarse_chan_bits=coarse_chan_bits, parallel_bits=parallel_coarse_streams, fine_bits=fine_fft_bits}
      mask prompts: coarse_chan_bits "Coarse FFT chans (2^?):"; parallel_bits "Parallel coarse chans (2^?):"; fine_bits "Fine FFT bits (2^?):"
      mask init:
      | fft_length = sprintf('%i', 2^fine_bits);
      | set_param([gcb, '/fft_pol0'], 'transform_length', fft_length);
      | set_param([gcb, '/fft_pol1'], 'transform_length', fft_length);
  sync_out : Outport
  data_out : Outport  Port=2
  fft_dv : Outport  Port=3
  data_index : Outport  Port=4
  fft_or0 : Outport  Port=5
  fft_or1 : Outport  Port=6
  snap_128bit : Outport  Port=7
  snap_buffer72 : Outport  Port=8
  snap_pfb72 : Outport  Port=9
  wires:
  sync/1 -> [sync], buffer/1(sync)
  coarse_chan_sel/1 -> [coarse_chan_sel], buffer/3(target)
  tvg_en/1 -> [tvg_en]
  Convert2/1 -> Concat2/1
  Convert1/1 -> Concat2/2
  Concat2/1 -> Mux4/3
  xilinx_ffts/4(xk_index) -> [xk_index]
  [channel_index] -> Convert2/1
  xilinx_ffts/1(out_sync) -> Delay4/1
  xilinx_ffts/3(out_valid) -> Delay5/1
  Delay4/1 -> sync_out/1, [sync_out]
  Delay1/1 -> data_out/1
  Delay5/1 -> fft_dv/1, [dv_out]
  xilinx_ffts/2(out_data) -> Delay1/1, Delay2/1
  Delay6/1 -> data_index/1
  bus_expand1/1(msb_out2) -> pfb_fir_async1/3(pol1_in1)
  bus_expand1/2(lsb_out1) -> pfb_fir_async1/4(pol1_in2)
  pfb_fir_async1/3(pol1_out1) -> bus_create/1
  pfb_fir_async1/4(pol1_out2) -> bus_create/2
  buffer/2(data) -> bus_expand1/1(bus_in), bus_create2/2(in2)
  buffer/1(sync_out) -> pfb_fir_async1/1(sync), bus_create2/1(in1)
  buffer/3(dvalid) -> pfb_fir_async1/2(dv), bus_create2/3(in3)
  pfb_fir_async1/1(sync_out) -> xilinx_ffts/1(sync), bus_create1/1(in1)
  bus_create/1 -> xilinx_ffts/2(data), bus_create1/2(in2)
  pfb_fir_async1/2(dv_out) -> bus_create1/3(in3)
  [mrst] -> xilinx_ffts/3(mrst)
  mrst/1 -> [mrst], buffer/4(mrst)
  [tvg_en] -> Mux4/1
  Mux4/1 -> bus_create3/2(in2)
  [sync_out] -> bus_create3/1(in1)
  [dv_out] -> bus_create3/3(in3)
  bus_create3/1(bus_out) -> snap_128bit/1
  data/1 -> buffer/2(din)
  [channel_index] -> Delay6/1
  [channel_offset] -> Convert1/1
  bus_create1/1(bus_out) -> snap_buffer72/1
  bus_create2/1(bus_out) -> snap_pfb72/1
  fine_fft_shift/1 -> xilinx_ffts/4(fftshift)
  xilinx_ffts/5(fftor0) -> fft_or0/1
  xilinx_ffts/6(fftor1) -> fft_or1/1
  Convert6/1 -> Mux4/2
  [coarse_chan_sel] -> indexgen/1(coarse_chan)
  [xk_index] -> indexgen/2(xk_index)
  indexgen/1(index) -> [channel_index]
  indexgen/2(offset) -> [channel_offset]
  Delay2/1 -> Convert6/1
